simulink model "Example_Getting_Started_UDP"  (R2016b)
settings: configuration reference "AR_Drone_ConfigSet" (kept outside this file)
libraries: AR_Drone_Sensors x1
settings Model: DataDictionary=ArDroneDataDictionary.sldd  SimulationMode=external  Creator=sannem  LastModifiedBy=SCBR
settings ConfigSetRef: DDName=ArDroneDataDictionary.sldd

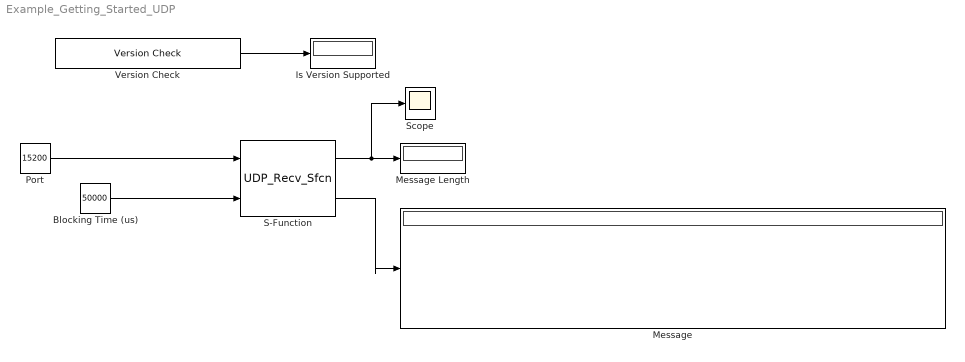
== system Example_Getting_Started_UDP ==
  Blocking Time (us) : Constant  Value=50000  OutDataTypeStr=double
  Is Version Supported : Display
  Message : Display
  Message Length : Display
  Port : Constant  Value=15200  OutDataTypeStr=int32
  S-Function : S-Function  FunctionName=UDP_Recv_Sfcn  Parameters=0.2  SFunctionDeploymentMode=off  EnableBusSupport=off
  Scope : Scope
  Version Check : AR_Drone_Sensors/Version Check  SFunctionSpec=void versionCheckStep(uint8 y1[1])  ShowSpec=off
  wires:
  Version Check/1 -> Is Version Supported/1
  S-Function/1 -> Scope/1, Message Length/1
  Port/1 -> S-Function/1
  S-Function/2 -> Message/1
  Blocking Time (us)/1 -> S-Function/2
